simulink model "state_space_simu"  (R2018b)
settings: Solver=VariableStepAuto  StartTime=0.0  StopTime=10.0  RelTol=1e-3
values from neighbouring files (symbols this model uses):
  A = [0 1; (g*m*l*cos(lp))/I -b/I]    [porte1.m]    (also in test.m)
  B = [0; 1/I]    [porte1.m]    (also in test.m)
  C = [1 0]    [porte1.m]    (also in test.m)
settings Model: Creator=Batman  LastModifiedBy=Batman

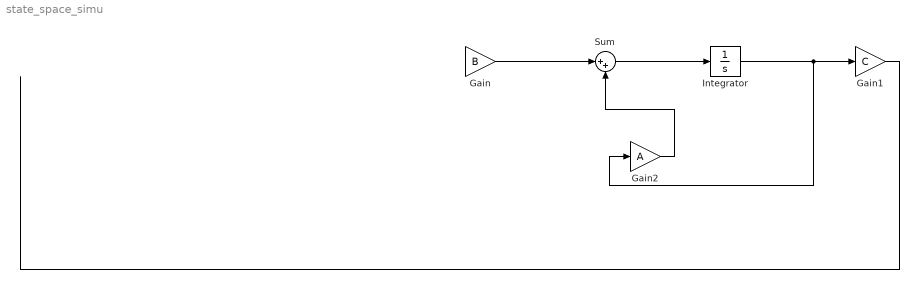
== system state_space_simu ==
  Gain : Gain  Gain=B
  Gain1 : Gain  Gain=C
  Gain2 : Gain  Gain=A
  Integrator : Integrator
  Sum : Sum  Inputs=|++
  wires:
  Integrator/1 -> Gain2/1, Gain1/1
  Sum/1 -> Integrator/1
  ? -> Gain/1
  Gain1/1 -> ?
  Gain/1 -> Sum/1
  Gain2/1 -> Sum/2
